simulink model "model_2"  (R2023a)
settings: Solver=VariableStepAuto  StartTime=0.0  StopTime=12  RelTol=1e-3
InitFcn:
  | init_const;
values from neighbouring files (symbols this model uses):
  D_l = [l_d1 0 ... (first row only)    [init_const.m]
  D_m = [m_d1 0 ... (first row only)    [init_const.m]
  g = 9.81    [init_const.m]
  J = [I1 0 ... (first row only)    [init_const.m]
  K = [k1 0 ... (first row only)    [init_const.m]
  l1 = 0.4    [init_const.m]
  l2 = 0.3    [init_const.m]
  m1 = 1    [init_const.m]
  m2 = 1    [init_const.m]
libraries: slpidlib x1, robotcorelib x1
settings Model: Creator=iqbal  LastModifiedBy=sabir
settings DebuggingCC: UnconnectedInputMsg=warning  UnconnectedOutputMsg=warning  UnconnectedLineMsg=warning
settings ModelReferenceCC: EnableRefExpFcnMdlSchedulingChecks=on
settings RTWCC: DLArmComputeVersion=19.05

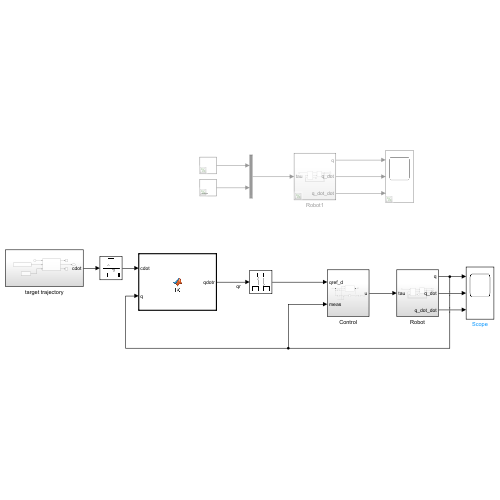
[thumbnail: Simulink's stored preview of the top-level diagram]
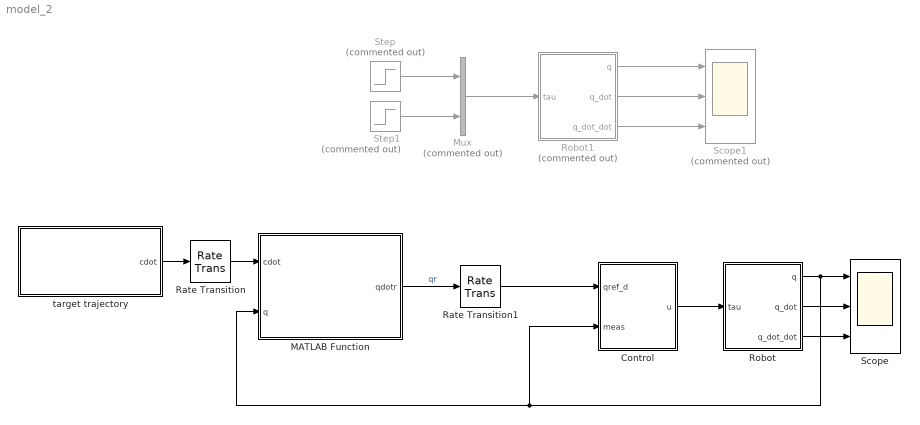
== system model_2 ==
  Control : Subsystem
  MATLAB Function : MATLAB Function  TreatAsAtomicUnit=on
  Mux : Mux  Commented=on  Inputs=2
  Rate Transition : RateTransition
  Rate Transition1 : RateTransition
  Robot : Subsystem
  Robot1 : Subsystem  Commented=on
  Scope : Scope  NumInputPorts=3
  Scope1 : Scope  Commented=on  NumInputPorts=3
  Step : Step  Commented=on  SampleTime=0
  Step1 : Step  Commented=on  SampleTime=0
  target trajectory : Subsystem
  wires:
  Robot/2(q_dot) -> Scope/2
  Robot/3(q_dot_dot) -> Scope/3
  Control/1(u) -> Robot/1(tau)
  MATLAB Function/1(qdotr) -> Rate Transition1/1  "qr"
  Robot/1(q) -> Scope/1, Control/2(meas), MATLAB Function/2(q)
  Rate Transition/1 -> MATLAB Function/1(cdot)
  target trajectory/1(cdot) -> Rate Transition/1
  Rate Transition1/1 -> Control/1(qref_d)
  Step/1 -> Mux/1
  Step1/1 -> Mux/2
  Mux/1 -> Robot1/1(tau)
  Robot1/1(q) -> Scope1/1
  Robot1/2(q_dot) -> Scope1/2
  Robot1/3(q_dot_dot) -> Scope1/3

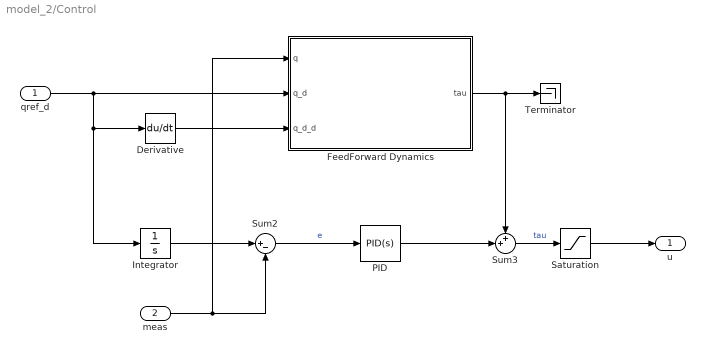
== system model_2/Control ==
  qref_d : Inport
  meas : Inport  Port=2
  Derivative : Derivative
  FeedForward Dynamics : MATLAB Function  TreatAsAtomicUnit=on
  Integrator : Integrator
  PID : slpidlib/PID Controller  Controller=PID  Form=Parallel  TimeDomain=Continuous-time  UseExternalTs=off  SampleTime=-1  IntegratorMethod=Forward Euler  FilterMethod=Forward Euler  ControllerParametersSource=internal  P=[25;18]  I=[4;3]  UseKiTs=off  D=[0.25;0.25]  N=700  UseFilter=on  TunerSelectOption=Transfer Function Based (PID Tuner App)  InitialConditionSource=internal  InitialConditionForIntegrator=0  InitialConditionForFilter=0  DifferentiatorICPrevScaledInput=0  ExternalReset=none  TrackingMode=off  Kt=1  LimitOutput=off  SatLimitsSource=internal  UpperSaturationLimit=inf  LowerSaturationLimit=-inf  LinearizeAsGain=on  AntiWindupMode=none  Kb=1  LimitIntegrator=off  UpperIntegratorSaturationLimit=inf  LowerIntegratorSaturationLimit=-inf  POutMin=[]  POutMax=[]  IOutMin=[]  IOutMax=[]  DOutMin=[]  DOutMax=[]  NOutMin=[]  NOutMax=[]  SumOutMin=[]  SumOutMax=[]  SaturationOutMin=[]  SaturationOutMax=[]  PParamMin=[]  PParamMax=[]  IParamMin=[]  IParamMax=[]  DParamMin=[]  DParamMax=[]  NParamMin=[]  NParamMax=[]  KbParamMin=[]  KbParamMax=[]  KtParamMin=[]  KtParamMax=[]  KbOutMin=[]  KbOutMax=[]  KtOutMin=[]  KtOutMax=[]  IntegratorOutMin=[]  IntegratorOutMax=[]  FilterOutMin=[]  FilterOutMax=[]  SumI1OutMin=[]  SumI1OutMax=[]  SumI2OutMin=[]  SumI2OutMax=[]  SumI3OutMin=[]  SumI3OutMax=[]  SumI4OutMin=[]  SumI4OutMax=[]  SumDOutMin=[]  SumDOutMax=[]  DifferentiatorOutMin=[]  DifferentiatorOutMax=[]  FilterDiffOutCoefMin=[]  FilterDiffOutCoefMax=[]  ReciprocalOutMin=[]  ReciprocalOutMax=[]  SumDenOutMin=[]  SumDenOutMax=[]  SumNumOutMin=[]  SumNumOutMax=[]  DivideOutMin=[]  DivideOutMax=[]  UdiffTsProdOutMin=[]  UdiffTsProdOutMax=[]  NTsProdOutMin=[]  NTsProdOutMax=[]  UintegralTsProdOutMin=[]  UintegralTsProdOutMax=[]  UngainTsProdOutMin=[]  UngainTsProdOutMax=[]  ClampingZeroOutDataTypeStr=Inherit: Inherit via back propagation  ClampingZeroOutMin=[]  ClampingZeroOutMax=[]  FilterDenConstantOutDataTypeStr=Inherit: Inherit via back propagation  FilterDenConstantOutMin=[]  FilterDenConstantOutMax=[]  PCopyOutDataTypeStr=Inherit: Inherit via back propagation  PCopyOutMin=[]  PCopyOutMax=[]  NCopyOutDataTypeStr=Inherit: Inherit via back propagation  NCopyOutMin=[]  NCopyOutMax=[]  IntegratorContinuousStateAttributes=''  IntegratorStateMustResolveToSignalObject=off  IntegratorRTWStateStorageClass=Auto  FilterContinuousStateAttributes=''  FilterStateMustResolveToSignalObject=off  FilterRTWStateStorageClass=Auto  ParallelPVariant=InternalParameters  IdealPVariant=Disabled  IVariant=InternalParameters  DVariant=InternalParameters  IntegratorVariant=Continuous  SatVariant=Disabled  AWVariant=Passthrough  PCopyVariant=Disabled  TRVariant=Disabled  FdbkBlocksVariant=Forward  IdealPFdbkVariant=Disabled  SatFdbkVariant=Disabled  DerivativeFilterVariant=ContFilter  NVariant=InternalParameters  NCopyVariant=Disabled  FilterICVariant=InternalICsFilter  IntegratorICVariant=InternalICs  ExternalResetVariant=Disabled  TRSumVariant=Passthrough  SumFdbkVariant=Disabled  SumVariant=Sum_PID  TsampFilterVariant=InternalTs  TsampNgainVariant=Passthrough  TsampIntegralVariant=Disabled_SignalSpec  ExternalSaturationOutDataTypeStr=Inherit: Same as second input
  Saturation : Saturate  UpperLimit=12  LowerLimit=-12
  Sum2 : Sum  Inputs=|+-
  Sum3 : Sum  Inputs=++|
  Terminator : Terminator
  u : Outport
  wires:
  meas/1 -> FeedForward Dynamics/1(q), Sum2/2
  Sum3/1 -> Saturation/1  "tau"
  PID/1 -> Sum3/2
  FeedForward Dynamics/1(tau) -> Sum3/1, Terminator/1
  Sum2/1 -> PID/1  "e"
  Saturation/1 -> u/1
  qref_d/1 -> Derivative/1, Integrator/1, FeedForward Dynamics/2(q_d)
  Derivative/1 -> FeedForward Dynamics/3(q_d_d)
  Integrator/1 -> Sum2/1

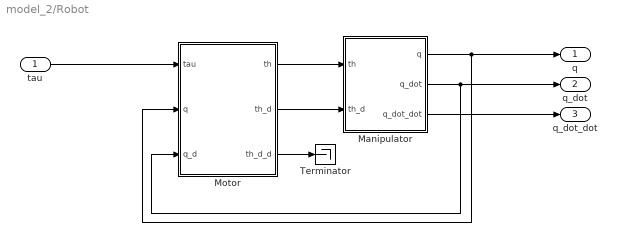
== system model_2/Robot ==
  tau : Inport
  Manipulator : Subsystem
  Motor : Subsystem
  Terminator : Terminator
  q : Outport
  q_dot : Outport  Port=2
  q_dot_dot : Outport  Port=3
  wires:
  Manipulator/2(q_dot) -> q_dot/1, Motor/3(q_d)
  Motor/2(th_d) -> Manipulator/2(th_d)
  Motor/3(th_d_d) -> Terminator/1
  Manipulator/1(q) -> q/1, Motor/2(q)
  Motor/1(th) -> Manipulator/1(th)
  Manipulator/3(q_dot_dot) -> q_dot_dot/1
  tau/1 -> Motor/1(tau)

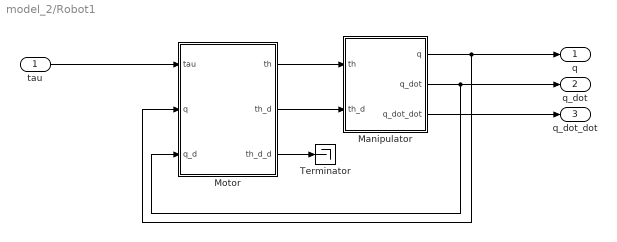
== system model_2/Robot1 ==
  tau : Inport
  Manipulator : Subsystem
  Motor : Subsystem
  Terminator : Terminator
  q : Outport
  q_dot : Outport  Port=2
  q_dot_dot : Outport  Port=3
  wires:
  tau/1 -> Motor/1(tau)
  Manipulator/3(q_dot_dot) -> q_dot_dot/1
  Motor/1(th) -> Manipulator/1(th)
  Manipulator/1(q) -> Motor/2(q), q/1
  Motor/3(th_d_d) -> Terminator/1
  Motor/2(th_d) -> Manipulator/2(th_d)
  Manipulator/2(q_dot) -> Motor/3(q_d), q_dot/1

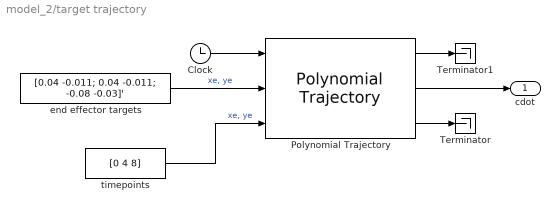
== system model_2/target trajectory ==
  Clock : Clock
  Polynomial Trajectory : robotcorelib/Polynomial Trajectory  WaypointSource=External  Waypoints=[ 0, 2, 1, 5, 0; -1, 3, 1, 4, 4 ]  TimePoints=[ 0, 1, 2, 3, 4 ]  TimeInterval=[ 1, 4 ]  Method=Cubic Polynomial  ParameterSource=Internal  VelocityBoundaryCondition=zeros( 2, 3 )  AccelerationBoundaryCondition=zeros( 2, 5 )  SimulateUsing=Interpreted execution
  Terminator : Terminator
  Terminator1 : Terminator
  end effector targets : Constant  Value=[0.04 -0.011; 0.04 -0.011; -0.08 -0.03]'
  timepoints : Constant  Value=[0 4 8]
  cdot : Outport
  wires:
  end effector targets/1 -> Polynomial Trajectory/2  "xe, ye"
  timepoints/1 -> Polynomial Trajectory/3  "xe, ye"
  Clock/1 -> Polynomial Trajectory/1
  Polynomial Trajectory/3 -> Terminator/1
  Polynomial Trajectory/2 -> cdot/1
  Polynomial Trajectory/1 -> Terminator1/1

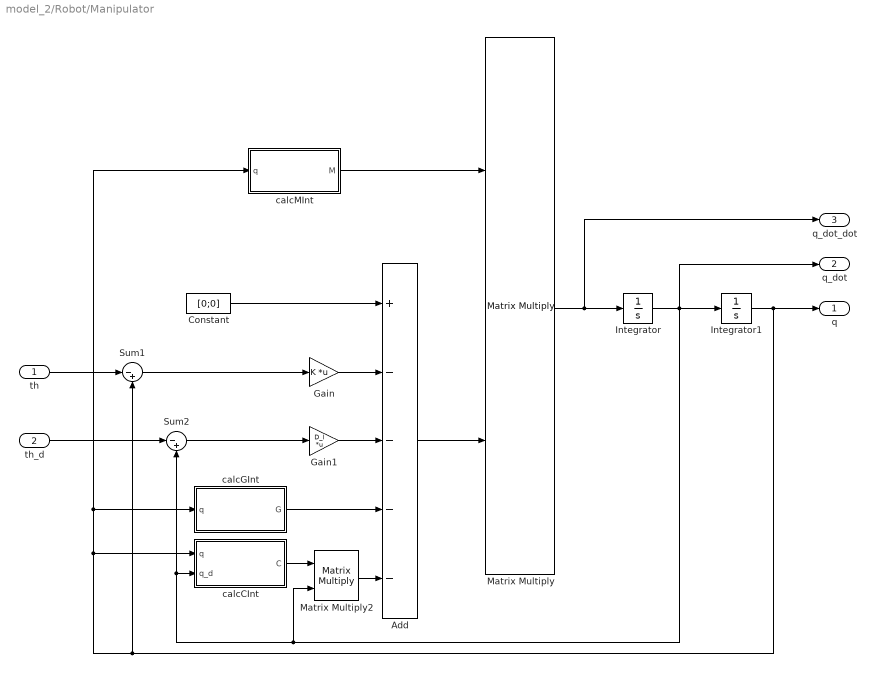
== system model_2/Robot/Manipulator ==
  th : Inport
  th_d : Inport  Port=2
  Add : Sum  Inputs=+----
  Constant : Constant  Value=[0;0]
  Gain : Gain  Gain=K  Multiplication=Matrix(K*u)
  Gain1 : Gain  Gain=D_l  Multiplication=Matrix(K*u)
  Integrator : Integrator
  Integrator1 : Integrator
  Matrix Multiply : Product  Multiplication=Matrix(*)
  Matrix Multiply2 : Product  Multiplication=Matrix(*)
  Sum1 : Sum  Inputs=|-+
  Sum2 : Sum  Inputs=|-+
  calcCInt : MATLAB Function  TreatAsAtomicUnit=on
  calcGInt : MATLAB Function  TreatAsAtomicUnit=on
  calcMInt : MATLAB Function  TreatAsAtomicUnit=on
  q : Outport
  q_dot : Outport  Port=2
  q_dot_dot : Outport  Port=3
  wires:
  Constant/1 -> Add/1
  Sum1/1 -> Gain/1
  Gain/1 -> Add/2
  Sum2/1 -> Gain1/1
  Gain1/1 -> Add/3
  Add/1 -> Matrix Multiply/2
  calcMInt/1(M) -> Matrix Multiply/1
  Matrix Multiply/1 -> q_dot_dot/1, Integrator/1
  Integrator/1 -> Matrix Multiply2/2, calcCInt/2(q_d), Sum2/2, q_dot/1, Integrator1/1
  Integrator1/1 -> Sum1/2, calcMInt/1(q), calcGInt/1(q), calcCInt/1(q), q/1
  th_d/1 -> Sum2/1
  th/1 -> Sum1/1
  calcGInt/1(G) -> Add/4
  Matrix Multiply2/1 -> Add/5
  calcCInt/1(C) -> Matrix Multiply2/1

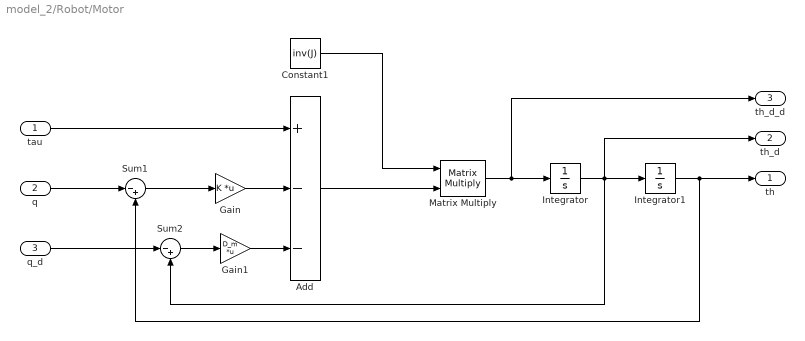
== system model_2/Robot/Motor ==
  tau : Inport
  q : Inport  Port=2
  q_d : Inport  Port=3
  Add : Sum  Inputs=+--
  Constant1 : Constant  Value=inv(J)
  Gain : Gain  Gain=K  Multiplication=Matrix(K*u)
  Gain1 : Gain  Gain=D_m  Multiplication=Matrix(K*u)
  Integrator : Integrator
  Integrator1 : Integrator
  Matrix Multiply : Product  Multiplication=Matrix(*)
  Sum1 : Sum  Inputs=|-+
  Sum2 : Sum  Inputs=|-+
  th : Outport
  th_d : Outport  Port=2
  th_d_d : Outport  Port=3
  wires:
  tau/1 -> Add/1
  q/1 -> Sum1/1
  Integrator/1 -> th_d/1, Sum2/2, Integrator1/1
  Gain/1 -> Add/2
  Gain1/1 -> Add/3
  Sum2/1 -> Gain1/1
  Add/1 -> Matrix Multiply/2
  Matrix Multiply/1 -> th_d_d/1, Integrator/1
  Sum1/1 -> Gain/1
  Constant1/1 -> Matrix Multiply/1
  q_d/1 -> Sum2/1
  Integrator1/1 -> th/1, Sum1/2

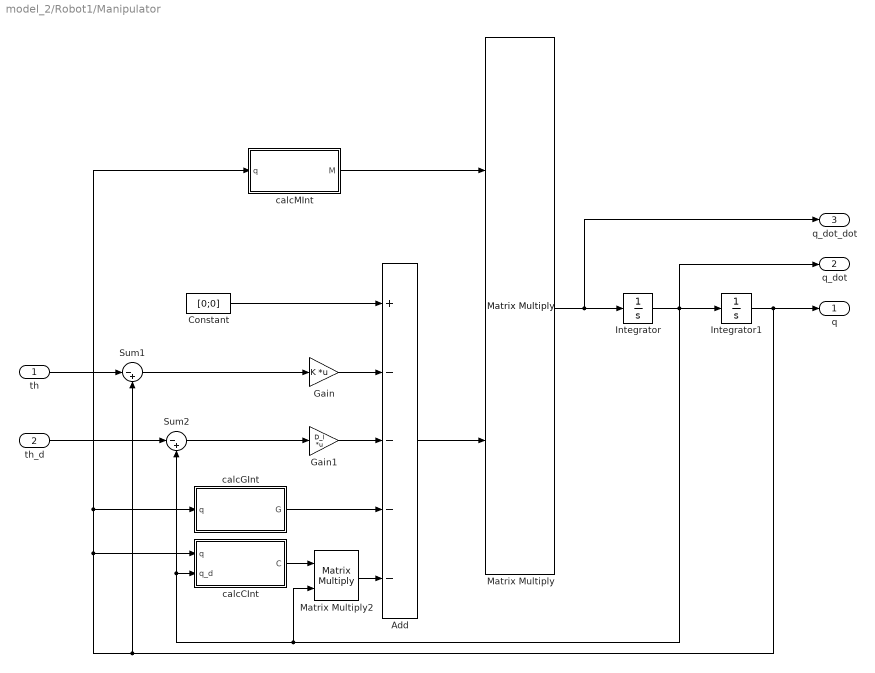
== system model_2/Robot1/Manipulator ==
  th : Inport
  th_d : Inport  Port=2
  Add : Sum  Inputs=+----
  Constant : Constant  Value=[0;0]
  Gain : Gain  Gain=K  Multiplication=Matrix(K*u)
  Gain1 : Gain  Gain=D_l  Multiplication=Matrix(K*u)
  Integrator : Integrator
  Integrator1 : Integrator
  Matrix Multiply : Product  Multiplication=Matrix(*)
  Matrix Multiply2 : Product  Multiplication=Matrix(*)
  Sum1 : Sum  Inputs=|-+
  Sum2 : Sum  Inputs=|-+
  calcCInt : MATLAB Function  TreatAsAtomicUnit=on
  calcGInt : MATLAB Function  TreatAsAtomicUnit=on
  calcMInt : MATLAB Function  TreatAsAtomicUnit=on
  q : Outport
  q_dot : Outport  Port=2
  q_dot_dot : Outport  Port=3
  wires:
  calcCInt/1(C) -> Matrix Multiply2/1
  Matrix Multiply2/1 -> Add/5
  calcGInt/1(G) -> Add/4
  th/1 -> Sum1/1
  th_d/1 -> Sum2/1
  Integrator1/1 -> q/1, calcCInt/1(q), calcGInt/1(q), calcMInt/1(q), Sum1/2
  Integrator/1 -> Integrator1/1, q_dot/1, Sum2/2, calcCInt/2(q_d), Matrix Multiply2/2
  Matrix Multiply/1 -> Integrator/1, q_dot_dot/1
  calcMInt/1(M) -> Matrix Multiply/1
  Add/1 -> Matrix Multiply/2
  Gain1/1 -> Add/3
  Sum2/1 -> Gain1/1
  Gain/1 -> Add/2
  Sum1/1 -> Gain/1
  Constant/1 -> Add/1

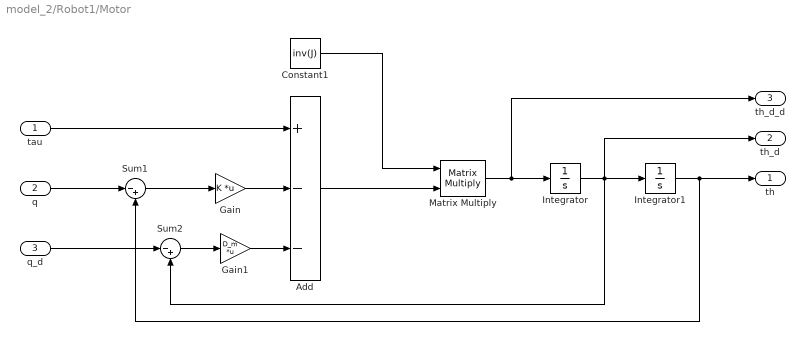
== system model_2/Robot1/Motor ==
  tau : Inport
  q : Inport  Port=2
  q_d : Inport  Port=3
  Add : Sum  Inputs=+--
  Constant1 : Constant  Value=inv(J)
  Gain : Gain  Gain=K  Multiplication=Matrix(K*u)
  Gain1 : Gain  Gain=D_m  Multiplication=Matrix(K*u)
  Integrator : Integrator
  Integrator1 : Integrator
  Matrix Multiply : Product  Multiplication=Matrix(*)
  Sum1 : Sum  Inputs=|-+
  Sum2 : Sum  Inputs=|-+
  th : Outport
  th_d : Outport  Port=2
  th_d_d : Outport  Port=3
  wires:
  Integrator1/1 -> Sum1/2, th/1
  q_d/1 -> Sum2/1
  Constant1/1 -> Matrix Multiply/1
  Sum1/1 -> Gain/1
  Matrix Multiply/1 -> Integrator/1, th_d_d/1
  Add/1 -> Matrix Multiply/2
  Sum2/1 -> Gain1/1
  Gain1/1 -> Add/3
  Gain/1 -> Add/2
  Integrator/1 -> Integrator1/1, Sum2/2, th_d/1
  q/1 -> Sum1/1
  tau/1 -> Add/1

== matlab function model_2/Robot/Manipulator/calcCInt ==
  data: q input; q_d input; C output size=[2 2]; m1 parameter; m2 parameter; l1 parameter; l2 parameter
function C = calcCInt(q, q_d, m1, m2, l1, l2)
C=[-2*l1*l2*m2*sin(q(2))*q_d(2) -l1*l2*m2*sin(q(2))*q_d(2);
      l1*l2*m2*sin(q(2))*q_d(1) 0];
end

== matlab function model_2/Robot/Manipulator/calcMInt ==
  data: q input; M output size=[2 2]; m1 parameter; m2 parameter; l1 parameter; l2 parameter
function M = calcMInt(q, m1, m2, l1, l2)
M=[(m1+m2)*l1^2+m2*l2^2+2*m2*l1*l2*cos(q(2)) m2*l2^2+m2*l1*l2*cos(q(2));
      m2*l2^2+m2*l1*l2*cos(q(2)) m2*l2^2];
M=inv(M);
end

== matlab function model_2/Robot/Manipulator/calcGInt ==
  data: q input; G output size=[2 1]; m1 parameter; m2 parameter; g parameter; l1 parameter; l2 parameter
function G = calcGInt(q, m1, m2, g, l1, l2)
G = -[(m1+m2)*g*l1*sin(q(1))+m2*g*l2*sin(q(1)+q(2));
         m2*g*l2*sin(q(1)+q(2))];
end

== matlab function model_2/MATLAB Function ==
  data: cdot input size=2; qdotr output size=2; l1 parameter; l2 parameter; q input size=2
function qdotr = IK(cdot, l1, l2, q)

q1 = q(1);
q2 = q(2);

Jfnc = @(L1,L2,q1,q2)reshape([-L2.*sin(q1+q2)-L1.*sin(q1),L2.*cos(q1+q2)+L1.*cos(q1),-L2.*sin(q1+q2),L2.*cos(q1+q2)],[2,2]);

J = Jfnc(l1,l2,q1,q2);

qdotr = pinv(J)*cdot;

end

== matlab function model_2/Robot1/Manipulator/calcCInt ==
  data: q input; q_d input; C output size=[2 2]; m1 parameter; m2 parameter; l1 parameter; l2 parameter
function C = calcCInt(q, q_d, m1, m2, l1, l2)
C=[-2*l1*l2*m2*sin(q(2))*q_d(2) -l1*l2*m2*sin(q(2))*q_d(2);
      l1*l2*m2*sin(q(2))*q_d(1) 0];
end

== matlab function model_2/Robot1/Manipulator/calcGInt ==
  data: q input; G output size=[2 1]; m1 parameter; m2 parameter; g parameter; l1 parameter; l2 parameter
function G = calcGInt(q, m1, m2, g, l1, l2)
G = -[(m1+m2)*g*l1*sin(q(1))+m2*g*l2*sin(q(1)+q(2));
         m2*g*l2*sin(q(1)+q(2))];
end

== matlab function model_2/Robot1/Manipulator/calcMInt ==
  data: q input; M output size=[2 2]; m1 parameter; m2 parameter; l1 parameter; l2 parameter
function M = calcMInt(q, m1, m2, l1, l2)
M=[(m1+m2)*l1^2+m2*l2^2+2*m2*l1*l2*cos(q(2)) m2*l2^2+m2*l1*l2*cos(q(2));
      m2*l2^2+m2*l1*l2*cos(q(2)) m2*l2^2];
M=inv(M);
end

== matlab function model_2/Control/FeedForward Dynamics ==
  data: q input size=2; tau output size=2; q_d input size=2; q_d_d input size=2; m1 parameter; m2 parameter; l1 parameter; l2 parameter; g parameter
function tau = ID(q, q_d, q_d_d, m1, m2, l1, l2, g)

q1 = q(1);
q2 = q(2);

q1dot = q_d(1);
q2dot = q_d(2);

M11 = (m1+m2)*l1^2 + m2*l2^2 + 2*m2*l1*l2*cos(q2);
M12 = m2*l2^2 + m2*l1*l2*cos(q2);
M21 = m2*l2^2+m2*l1*l2*cos(q2);
M22 = m2*l2^2;

M = [M11 M12; ...
     M21 M22];

C11 = -m2*l1*l2*2*q2dot*sin(q2);
C12 = -m2*l1*l2*q2dot*sin(q2); 

C21 = m2*l1*l2*q1dot*sin(q2);
C22 = 0;

C = [C11 C12; ...
     C21 C22];

tauG1 = (m1+m2)*g*l1*sin(q1) + m2*g*l2*sin(q1+q2);
tauG2 = m2*g*l2*sin(q1+q2);

tauG = [tauG1;...
        tauG2];



tau = M*q_d_d + C*q_d + tauG + [0.3 0;0 0.3]*q_d;

end
